simulink model "controller_estimator_test_static"  (R2016b)
settings: Solver=FixedStepAuto  StartTime=0.0  StopTime=5400  MaxStep=0.005  RelTol=1e-3
values from neighbouring files (symbols this model uses):
  quat_cmd = quat_cmd/norm(quat_cmd)    [controller_estimator_test_init.m]    (also in ctrl_est_test.m)
  sun_vec_init = sun_vec_init/norm(sun_vec_init)    [controller_estimator_test_init.m]    (also in ctrl_est_test.m)
undefined symbols (not defined in the file or in its folder): DiscIntNeverNeededParam, sim_params
libraries: aerolibutil x3, extended_kalman_filter_lib x1, pd_control_lib x1, vrlib x1, sensor_processing_libs x1, gyroscope_lib x1, mag_vec_LS_lib x1, dynamics_lib x1
settings Model: Creator=sexymathemagician  LastModifiedBy=Taylor

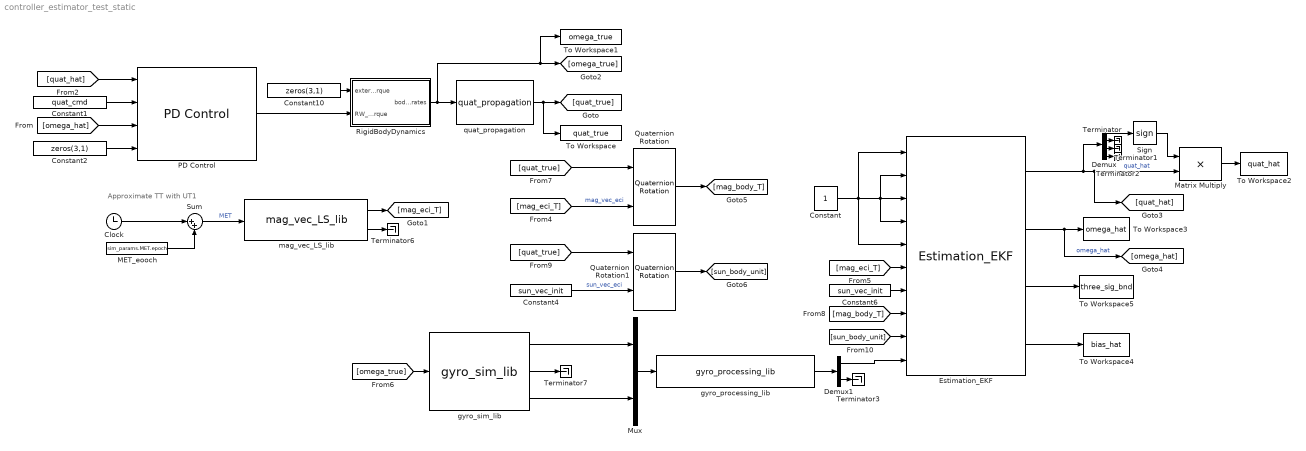
== system controller_estimator_test_static ==
  note: Approximate TT with UT1
  Clock : Clock
  Constant : Constant
  Constant1 : Constant  Value=quat_cmd
  Constant10 : Constant  Value=zeros(3,1)
  Constant2 : Constant  Value=zeros(3,1)
  Constant4 : Constant  Value=sun_vec_init
  Constant6 : Constant  Value=sun_vec_init
  Demux : Demux
  Demux1 : Demux  Outputs=[3 1]
  "Estimation_EKF " : extended_kalman_filter_lib/Estimation_EKF 
  MET_eooch : Constant  Value=sim_params.MET.epoch
  Matrix Multiply : Product
  Mux : Mux  Inputs=[3 1]
  PD Control : pd_control_lib/PD Control
  Quaternion Rotation : aerolibutil/Quaternion Rotation
  Quaternion Rotation1 : aerolibutil/Quaternion Rotation
  RigidBodyDynamics : Subsystem  AncestorBlock=dynamics_lib/Dynamics/RigidBodyDynamics
  Sign : Signum
  Sum : Sum  Inputs=|++
  Terminator{,1..3,6..7} (6 alike) : Terminator
  To Workspace : ToWorkspace  VariableName=quat_true  SaveFormat=Timeseries  SampleTime=-1
  To Workspace1 : ToWorkspace  VariableName=omega_true  SaveFormat=Timeseries  SampleTime=-1
  To Workspace2 : ToWorkspace  VariableName=quat_hat  SaveFormat=Timeseries  SampleTime=-1
  To Workspace3 : ToWorkspace  VariableName=omega_hat  SaveFormat=Timeseries  SampleTime=-1
  To Workspace4 : ToWorkspace  VariableName=bias_hat  SaveFormat=Timeseries  SampleTime=-1
  To Workspace5 : ToWorkspace  VariableName=three_sig_bnd  SaveFormat=Timeseries  SampleTime=-1
  gyro_processing_lib : sensor_processing_libs/gyro_processing_lib
  gyro_sim_lib : gyroscope_lib/gyro_sim_lib
  mag_vec_LS_lib : mag_vec_LS_lib/mag_vec_LS_lib
  quat_propagation : dynamics_lib/Dynamics/quat_propagation
  wires:
  Constant/1 -> "Estimation_EKF "/5, "Estimation_EKF "/1, "Estimation_EKF "/4, "Estimation_EKF "/2, "Estimation_EKF "/3
  "Estimation_EKF "/3 -> To Workspace5/1
  "Estimation_EKF "/4 -> To Workspace4/1
  "Estimation_EKF "/2 -> [omega_hat], To Workspace3/1  "omega_hat"
  "Estimation_EKF "/1 -> Demux/1, [quat_hat], Matrix Multiply/2  "quat_hat"
  Demux/2 -> Terminator/1
  Demux/3 -> Terminator1/1
  Demux/4 -> Terminator2/1
  Demux/1 -> Sign/1
  Sign/1 -> Matrix Multiply/1
  Constant4/1 -> Quaternion Rotation1/2  "sun_vec_eci"
  [mag_eci_T] -> Quaternion Rotation/2  "mag_vec_eci"
  Constant6/1 -> "Estimation_EKF "/7
  [mag_eci_T] -> "Estimation_EKF "/6
  Matrix Multiply/1 -> To Workspace2/1
  RigidBodyDynamics/1(body_rates) -> To Workspace1/1, [omega_true], quat_propagation/1
  PD Control/1 -> RigidBodyDynamics/2(RW_torque)
  Constant1/1 -> PD Control/2
  quat_propagation/1 -> To Workspace/1, [quat_true]
  Constant2/1 -> PD Control/4
  Constant10/1 -> RigidBodyDynamics/1(external_torque)
  Sum/1 -> mag_vec_LS_lib/1  "MET"
  Clock/1 -> Sum/1
  MET_eooch/1 -> Sum/2
  mag_vec_LS_lib/1 -> [mag_eci_T]
  mag_vec_LS_lib/2 -> Terminator6/1
  [quat_hat] -> PD Control/1
  [omega_hat] -> PD Control/3
  gyro_sim_lib/3 -> Mux/2
  gyro_sim_lib/2 -> Terminator7/1
  gyro_sim_lib/1 -> Mux/1
  [omega_true] -> gyro_sim_lib/1
  Mux/1 -> gyro_processing_lib/1
  [quat_true] -> Quaternion Rotation/1
  Quaternion Rotation/1 -> [mag_body_T]
  [mag_body_T] -> "Estimation_EKF "/8
  [quat_true] -> Quaternion Rotation1/1
  Quaternion Rotation1/1 -> [sun_body_unit]
  [sun_body_unit] -> "Estimation_EKF "/9
  gyro_processing_lib/1 -> Demux1/1
  Demux1/1 -> "Estimation_EKF "/10
  Demux1/2 -> Terminator3/1

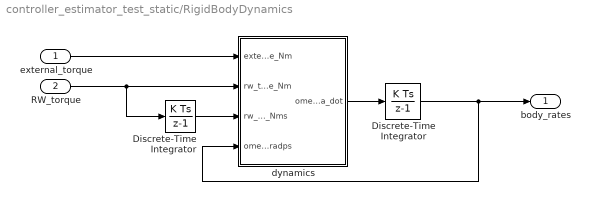
== system controller_estimator_test_static/RigidBodyDynamics ==
  external_torque : Inport
  RW_torque : Inport  Port=2
  Discrete-Time Integrator : DiscreteIntegrator  InitialCondition=fsw_params.control.cmd_processing.ic.momentum  InitialConditionSetting=State (most efficient)  SampleTime=-1  ICPrevOutput=DiscIntNeverNeededParam  ICPrevScaledInput=DiscIntNeverNeededParam
  "Discrete-Time Integrator " : DiscreteIntegrator  InitialCondition=sim_params.dynamics.ic.rate_init  InitialConditionSetting=State (most efficient)  SampleTime=-1  ICPrevOutput=DiscIntNeverNeededParam  ICPrevScaledInput=DiscIntNeverNeededParam
  dynamics : Subsystem
  body_rates : Outport
  wires:
  RW_torque/1 -> dynamics/2(rw_torque_Nm), Discrete-Time Integrator/1
  Discrete-Time Integrator/1 -> dynamics/3(rw_momentum_Nms)
  "Discrete-Time Integrator "/1 -> body_rates/1, dynamics/4(omega_radps)
  external_torque/1 -> dynamics/1(external_torque_Nm)
  dynamics/1(omega_dot) -> "Discrete-Time Integrator "/1

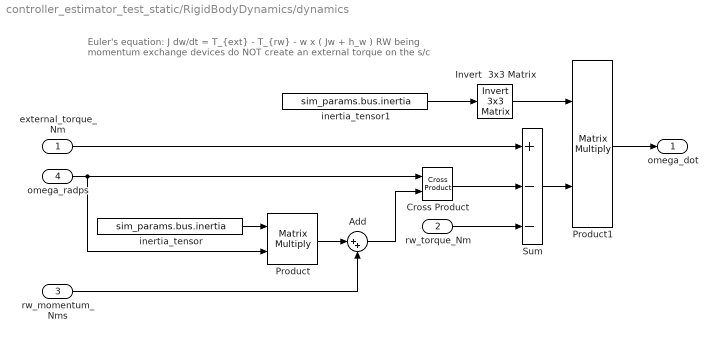
== system controller_estimator_test_static/RigidBodyDynamics/dynamics ==
  note: Euler's equation: J dw/dt = T_{ext} - T_{rw} - w x ( Jw + h_w )
      |
      | RW being momentum exchange devices do NOT create
      | an external torque on the s/c
  external_torque_Nm : Inport
  rw_torque_Nm : Inport  Port=2
  rw_momentum_Nms : Inport  Port=3
  omega_radps : Inport  Port=4
  Add : Sum  Inputs=|++
  Cross Product : vrlib/Utilities/Cross Product
  Invert  3x3 Matrix : aerolibutil/Invert  3x3 Matrix
  Product : Product  Multiplication=Matrix(*)  RndMeth=Zero
  Product1 : Product  Multiplication=Matrix(*)  RndMeth=Zero
  Sum : Sum  Inputs=+--
  inertia_tensor : Constant  Value=sim_params.bus.inertia  SampleTime=-1
  inertia_tensor1 : Constant  Value=sim_params.bus.inertia  SampleTime=sim_params.sample_time_s
  omega_dot : Outport
  wires:
  rw_torque_Nm/1 -> Sum/3
  Add/1 -> Cross Product/2
  rw_momentum_Nms/1 -> Add/2
  Product/1 -> Add/1
  Cross Product/1 -> Sum/2
  inertia_tensor1/1 -> Invert  3x3 Matrix/1
  Invert  3x3 Matrix/1 -> Product1/1
  Product1/1 -> omega_dot/1
  Sum/1 -> Product1/2
  inertia_tensor/1 -> Product/1
  omega_radps/1 -> Cross Product/1, Product/2
  external_torque_Nm/1 -> Sum/1
